simulink model "Final_IHA_2706_2015a"  (R2016b)
settings: Solver=ode5  StartTime=0.0  StopTime=20  FixedStep=SampleTime  RelTol=1e-3  EnableMultiTasking=on
values from neighbouring files (symbols this model uses):
  K = 2000    [code_final.m]
  PowerOn = 0    [code_final.m]
  q = 41.3    [code_final.m]
  Q_AT_break = [-1 -0.7 -0.5 -0.3 -0.2 -0.1 0 0.2 0.8 1]    [code_final.m]
  Q_AT_look = [1 0.1991 0.1227 0.07575 0.04002 0.01761 0.00075 5.86e-8 5.86e-8 5.86e-8]    [code_final.m]
  Q_BT_break = [-1 -0.6 -0.2 0 0.1 0.2 0.3 0.4 0.5 1]    [code_final.m]
  Q_BT_look = [5.86e-8 5.86e-8 5.86e-8 0.000913 0.02175 0.040 0.081 0.10 0.20 1]    [code_final.m]
  Q_PA_break = [-1 -0.6 -0.2 0 0.1 0.2 0.3 0.4 0.5 1]    [code_final.m]
  Q_PA_look = [5.86e-8 5.86e-8 5.86e-8 0.000876 0.0214 0.044 0.071 0.1 0.15 1]    [code_final.m]
  Q_PB_break = [-1 -0.7 -0.5 -0.3 -0.2 -0.1 0 0.2 0.8 1]    [code_final.m]
  Q_PB_look = [1 0.1498 0.1 0.077 0.03591 0.021 0.00082 5.86e-8 5.86e-8 5.86e-8]    [code_final.m]
  SampleTime = .001    (= 0.001)    [code_final.m]
undefined symbols (not defined in the file or in its folder): b, Cylinder, Cylinder1, Cylinder2, Cylinder3, Cylinder4, DiscIntNeverNeededParam, FC, FL1, FL2, FS, Lift, Pillar, Pinion, Piston, Rack, tilt, Valve, VS, X, X1, X2, Y, Z
undefined symbols (not defined in the file): Cyl, HoseA, HoseB, Valve2, Valve3, Valve4
libraries: sm_lib x67, simulink x32, nesl_utility x20, simulink_extras x3, xpcrtudplib x2, xpcobsoletelib x2
(part 3 of 4)

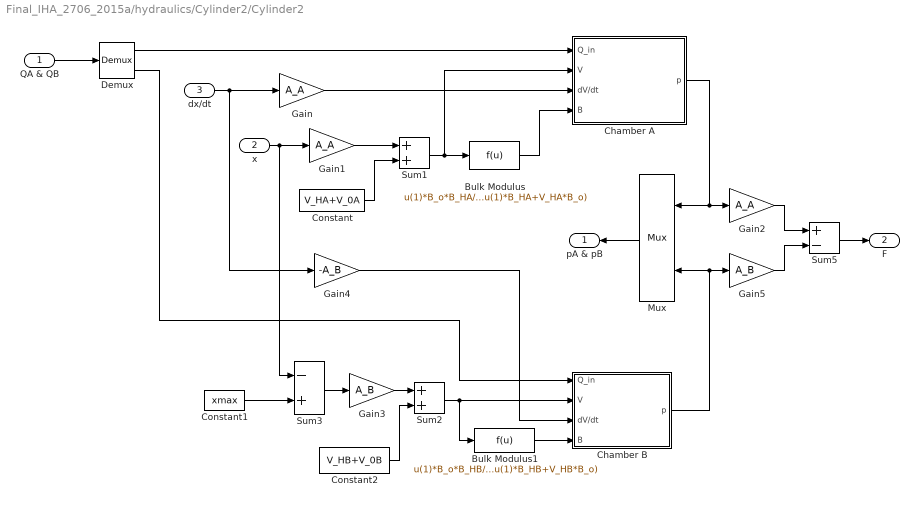
== system Final_IHA_2706_2015a/hydraulics/Cylinder2/Cylinder2 ==
  QA & QB : Inport
  x : Inport  Port=2
  dx/dt : Inport  Port=3
  Bulk Modulus : Fcn  Expr=u(1)*B_o*B_HA/(u(1)*B_HA+V_HA*B_o)
  Bulk Modulus1 : Fcn  Expr=u(1)*B_o*B_HB/(u(1)*B_HB+V_HB*B_o)
  Chamber A : Subsystem  mask(Hydraulic){pinitial=p_0A}
      mask prompts: pinitial "Initial pressure [Pa] :"
      mask help: Lumped fluid volume. Pressure is limited greater or equal to zero by saturation block corresponding to a rough model of cavitation.
      mask Help: eval('hydlibdoc(''vol_cav_doc'')')
  Chamber B : Subsystem  mask(Hydraulic){pinitial=p_0B}
      mask prompts: pinitial "Initial pressure [Pa] :"
      mask help: Lumped fluid volume. Pressure is limited greater or equal to zero by saturation block corresponding to a rough model of cavitation.
      mask Help: eval('hydlibdoc(''vol_cav_doc'')')
  Constant : Constant  Value=V_HA+V_0A
  Constant1 : Constant  Value=xmax
  Constant2 : Constant  Value=V_HB+V_0B
  Demux : Demux  Outputs=2
  Gain : Gain  Gain=A_A  SaturateOnIntegerOverflow=on  OutDataTypeStr=Inherit: Same as input  ParamDataTypeStr=Inherit: Same as input
  Gain1 : Gain  Gain=A_A  SaturateOnIntegerOverflow=on  OutDataTypeStr=Inherit: Same as input  ParamDataTypeStr=Inherit: Same as input
  Gain2 : Gain  Gain=A_A  SaturateOnIntegerOverflow=on  OutDataTypeStr=Inherit: Same as input  ParamDataTypeStr=Inherit: Same as input
  Gain3 : Gain  Gain=A_B  SaturateOnIntegerOverflow=on  OutDataTypeStr=Inherit: Same as input  ParamDataTypeStr=Inherit: Same as input
  Gain4 : Gain  Gain=-A_B  SaturateOnIntegerOverflow=on  OutDataTypeStr=Inherit: Same as input  ParamDataTypeStr=Inherit: Same as input
  Gain5 : Gain  Gain=A_B  SaturateOnIntegerOverflow=on  OutDataTypeStr=Inherit: Same as input  ParamDataTypeStr=Inherit: Same as input
  Mux : Mux  Inputs=2
  Sum1 : Sum  SaturateOnIntegerOverflow=on  InputSameDT=on  OutDataTypeStr=Inherit: Same as first input
  Sum2 : Sum  SaturateOnIntegerOverflow=on  InputSameDT=on  OutDataTypeStr=Inherit: Same as first input
  Sum3 : Sum  Inputs=-+  SaturateOnIntegerOverflow=on  InputSameDT=on  OutDataTypeStr=Inherit: Same as first input
  Sum5 : Sum  Inputs=+-  SaturateOnIntegerOverflow=on  InputSameDT=on  OutDataTypeStr=Inherit: Same as first input
  pA & pB : Outport  InitialOutput=0
  F : Outport  Port=2  InitialOutput=0
  wires:
  Constant/1 -> Sum1/2
  Sum1/1 -> Chamber A/2(" V"), Bulk Modulus/1
  Gain1/1 -> Sum1/1
  x/1 -> Gain1/1, Sum3/1
  QA & QB/1 -> Demux/1
  Chamber B/1(p) -> Gain5/1, Mux/2
  Sum5/1 -> F/1
  Gain5/1 -> Sum5/2
  Gain2/1 -> Sum5/1
  Chamber A/1(p) -> Gain2/1, Mux/1
  Mux/1 -> pA & pB/1
  Bulk Modulus/1 -> Chamber A/4(" B")
  Demux/1 -> Chamber A/1(Q_in)
  Bulk Modulus1/1 -> Chamber B/4(" B")
  Gain4/1 -> Chamber B/3(" dV/dt")
  Sum2/1 -> Chamber B/2(" V"), Bulk Modulus1/1
  Demux/2 -> Chamber B/1(Q_in)
  Constant1/1 -> Sum3/2
  Sum3/1 -> Gain3/1
  Gain3/1 -> Sum2/1
  Constant2/1 -> Sum2/2
  Gain/1 -> Chamber A/3(" dV/dt")
  dx/dt/1 -> Gain/1, Gain4/1

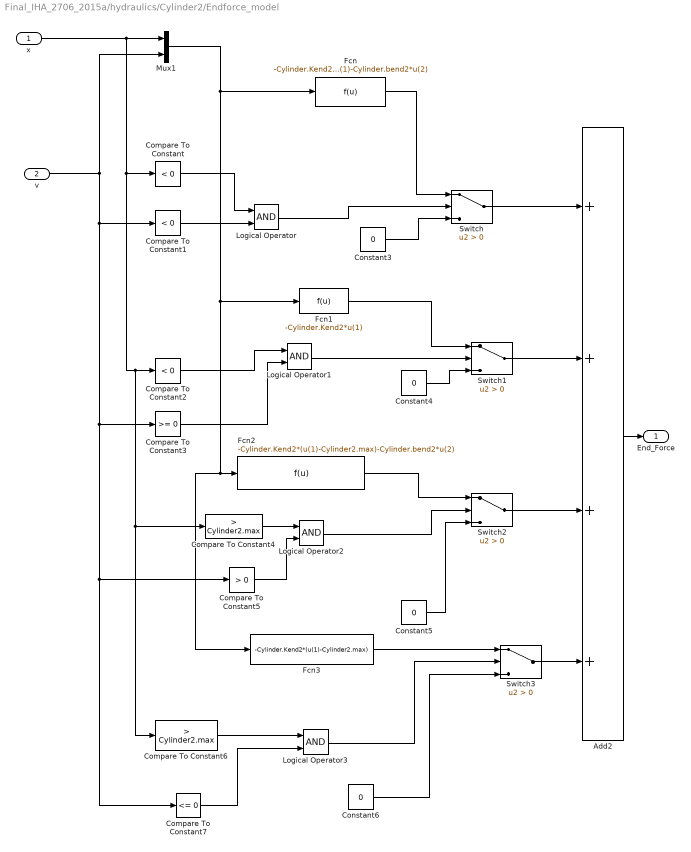
== system Final_IHA_2706_2015a/hydraulics/Cylinder2/Endforce_model ==
  x : Inport
  v : Inport  Port=2
  Add2 : Sum  Inputs=++++
  Compare To Constant : simulink/Logic and Bit Operations/Compare To Constant  relop=<  const=0  OutDataTypeStr=boolean
  Compare To Constant1 : simulink/Logic and Bit Operations/Compare To Constant  relop=<  const=0  OutDataTypeStr=boolean
  Compare To Constant2 : simulink/Logic and Bit Operations/Compare To Constant  relop=<  const=0  OutDataTypeStr=boolean
  Compare To Constant3 : simulink/Logic and Bit Operations/Compare To Constant  relop=>=  const=0  OutDataTypeStr=boolean
  Compare To Constant4 : simulink/Logic and Bit Operations/Compare To Constant  relop=>  const=Cylinder2.max  OutDataTypeStr=boolean
  Compare To Constant5 : simulink/Logic and Bit Operations/Compare To Constant  relop=>  const=0  OutDataTypeStr=boolean
  Compare To Constant6 : simulink/Logic and Bit Operations/Compare To Constant  relop=>  const=Cylinder2.max  OutDataTypeStr=boolean
  Compare To Constant7 : simulink/Logic and Bit Operations/Compare To Constant  relop=<=  const=0  OutDataTypeStr=boolean
  Constant{3..6} (4 alike) : Constant  Value=0
  Fcn : Fcn  Expr=-Cylinder.Kend2*u(1)-Cylinder.bend2*u(2)
  Fcn1 : Fcn  Expr=-Cylinder.Kend2*u(1)
  Fcn2 : Fcn  Expr=-Cylinder.Kend2*(u(1)-Cylinder2.max)-Cylinder.bend2*u(2)
  Fcn3 : Fcn  Expr=-Cylinder.Kend2*(u(1)-Cylinder2.max)
  Logical Operator{,1..3} (4 alike) : Logic  AllPortsSameDT=off  OutDataTypeStr=boolean
  Mux1 : Mux  Inputs=2
  Switch{,1..3} (4 alike) : Switch  Criteria=u2 > Threshold
  End_Force : Outport
  wires:
  x/1 -> Compare To Constant/1, Compare To Constant2/1, Compare To Constant4/1, Compare To Constant6/1, Mux1/1
  v/1 -> Compare To Constant1/1, Compare To Constant3/1, Compare To Constant5/1, Compare To Constant7/1, Mux1/2
  Fcn2/1 -> Switch2/1
  Logical Operator3/1 -> Switch3/2
  Fcn3/1 -> Switch3/1
  Compare To Constant5/1 -> Logical Operator2/2
  Switch2/1 -> Add2/3
  Constant6/1 -> Switch3/3
  Compare To Constant6/1 -> Logical Operator3/1
  Switch/1 -> Add2/1
  Constant5/1 -> Switch2/3
  Logical Operator2/1 -> Switch2/2
  Compare To Constant7/1 -> Logical Operator3/2
  Switch1/1 -> Add2/2
  Add2/1 -> End_Force/1
  Mux1/1 -> Fcn/1, Fcn3/1, Fcn2/1, Fcn1/1
  Switch3/1 -> Add2/4
  Compare To Constant2/1 -> Logical Operator1/1
  Compare To Constant1/1 -> Logical Operator/2
  Constant4/1 -> Switch1/3
  Logical Operator1/1 -> Switch1/2
  Fcn/1 -> Switch/1
  Logical Operator/1 -> Switch/2
  Constant3/1 -> Switch/3
  Compare To Constant/1 -> Logical Operator/1
  Compare To Constant4/1 -> Logical Operator2/1
  Fcn1/1 -> Switch1/1
  Compare To Constant3/1 -> Logical Operator1/2

== system Final_IHA_2706_2015a/hydraulics/Cylinder2/Friction_model ==
  v : Inport
  Add : Sum
  Fcn : Fcn  Expr=tanh(K*u)
  Fcn1 : Fcn  Expr=FC.c2+(FS.c2-FC.c2)*exp(-(u/VS.c2)^2)
  Fcn2 : Fcn  Expr=b.c2*u
  Product : Product
  Friction_Force : Outport
  wires:
  Fcn/1 -> Product/1
  Fcn1/1 -> Product/2
  Fcn2/1 -> Add/2
  Product/1 -> Add/1
  v/1 -> Fcn/1, Fcn2/1, Fcn1/1
  Add/1 -> Friction_Force/1

== system Final_IHA_2706_2015a/hydraulics/Cylinder2/Valve System2 ==
  p_A : Inport
  Uvalve : Inport  Port=2
  p_B : Inport  Port=3
  p_S : Inport  Port=4
  p_T : Inport  Port=5
  Flow paths : Subsystem
  Relative openings : Subsystem
  Scope : Scope
  Terminator1 : Terminator
  Terminator2 : Terminator
  Valve Dynamics : Subsystem
  Q_A : Outport
  Q_B : Outport  Port=2
  wires:
  p_A/1 -> Flow paths/5(p_A)
  p_T/1 -> Flow paths/8("p_T ")
  p_S/1 -> Flow paths/7(p_S)
  Flow paths/1(Q_A) -> Q_A/1, Scope/1
  p_B/1 -> Flow paths/6(p_B)
  Relative openings/1(av_PA) -> Flow paths/1(av_PA)
  Relative openings/3(av_BT) -> Flow paths/2(av_BT)
  Relative openings/4(av_AT) -> Flow paths/4(av_AT)
  Relative openings/2(av_PB) -> Flow paths/3(av_PB)
  Valve Dynamics/1(Spool Position [-1....1]) -> Relative openings/1(Spool_position)
  Flow paths/4(Q_T) -> Terminator2/1
  Flow paths/3(Q_P) -> Terminator1/1
  Flow paths/2(Q_B) -> Q_B/1
  Uvalve/1 -> Valve Dynamics/1(Control [-1....1])

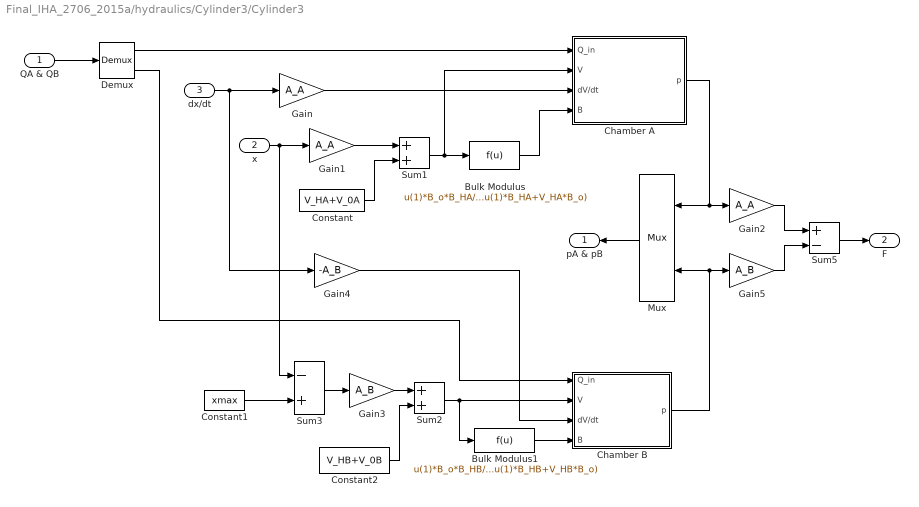
== system Final_IHA_2706_2015a/hydraulics/Cylinder3/Cylinder3 ==
  QA & QB : Inport
  x : Inport  Port=2
  dx/dt : Inport  Port=3
  Bulk Modulus : Fcn  Expr=u(1)*B_o*B_HA/(u(1)*B_HA+V_HA*B_o)
  Bulk Modulus1 : Fcn  Expr=u(1)*B_o*B_HB/(u(1)*B_HB+V_HB*B_o)
  Chamber A : Subsystem  mask(Hydraulic){pinitial=p_0A}
      mask prompts: pinitial "Initial pressure [Pa] :"
      mask help: Lumped fluid volume. Pressure is limited greater or equal to zero by saturation block corresponding to a rough model of cavitation.
      mask Help: eval('hydlibdoc(''vol_cav_doc'')')
  Chamber B : Subsystem  mask(Hydraulic){pinitial=p_0B}
      mask prompts: pinitial "Initial pressure [Pa] :"
      mask help: Lumped fluid volume. Pressure is limited greater or equal to zero by saturation block corresponding to a rough model of cavitation.
      mask Help: eval('hydlibdoc(''vol_cav_doc'')')
  Constant : Constant  Value=V_HA+V_0A
  Constant1 : Constant  Value=xmax
  Constant2 : Constant  Value=V_HB+V_0B
  Demux : Demux  Outputs=2
  Gain : Gain  Gain=A_A  SaturateOnIntegerOverflow=on  OutDataTypeStr=Inherit: Same as input  ParamDataTypeStr=Inherit: Same as input
  Gain1 : Gain  Gain=A_A  SaturateOnIntegerOverflow=on  OutDataTypeStr=Inherit: Same as input  ParamDataTypeStr=Inherit: Same as input
  Gain2 : Gain  Gain=A_A  SaturateOnIntegerOverflow=on  OutDataTypeStr=Inherit: Same as input  ParamDataTypeStr=Inherit: Same as input
  Gain3 : Gain  Gain=A_B  SaturateOnIntegerOverflow=on  OutDataTypeStr=Inherit: Same as input  ParamDataTypeStr=Inherit: Same as input
  Gain4 : Gain  Gain=-A_B  SaturateOnIntegerOverflow=on  OutDataTypeStr=Inherit: Same as input  ParamDataTypeStr=Inherit: Same as input
  Gain5 : Gain  Gain=A_B  SaturateOnIntegerOverflow=on  OutDataTypeStr=Inherit: Same as input  ParamDataTypeStr=Inherit: Same as input
  Mux : Mux  Inputs=2
  Sum1 : Sum  SaturateOnIntegerOverflow=on  InputSameDT=on  OutDataTypeStr=Inherit: Same as first input
  Sum2 : Sum  SaturateOnIntegerOverflow=on  InputSameDT=on  OutDataTypeStr=Inherit: Same as first input
  Sum3 : Sum  Inputs=-+  SaturateOnIntegerOverflow=on  InputSameDT=on  OutDataTypeStr=Inherit: Same as first input
  Sum5 : Sum  Inputs=+-  SaturateOnIntegerOverflow=on  InputSameDT=on  OutDataTypeStr=Inherit: Same as first input
  pA & pB : Outport  InitialOutput=0
  F : Outport  Port=2  InitialOutput=0
  wires:
  dx/dt/1 -> Gain4/1, Gain/1
  Gain/1 -> Chamber A/3(" dV/dt")
  Constant2/1 -> Sum2/2
  Gain3/1 -> Sum2/1
  Sum3/1 -> Gain3/1
  Constant1/1 -> Sum3/2
  Demux/2 -> Chamber B/1(Q_in)
  Sum2/1 -> Bulk Modulus1/1, Chamber B/2(" V")
  Gain4/1 -> Chamber B/3(" dV/dt")
  Bulk Modulus1/1 -> Chamber B/4(" B")
  Demux/1 -> Chamber A/1(Q_in)
  Bulk Modulus/1 -> Chamber A/4(" B")
  Mux/1 -> pA & pB/1
  Chamber A/1(p) -> Mux/1, Gain2/1
  Gain2/1 -> Sum5/1
  Gain5/1 -> Sum5/2
  Sum5/1 -> F/1
  Chamber B/1(p) -> Mux/2, Gain5/1
  QA & QB/1 -> Demux/1
  x/1 -> Sum3/1, Gain1/1
  Gain1/1 -> Sum1/1
  Sum1/1 -> Bulk Modulus/1, Chamber A/2(" V")
  Constant/1 -> Sum1/2

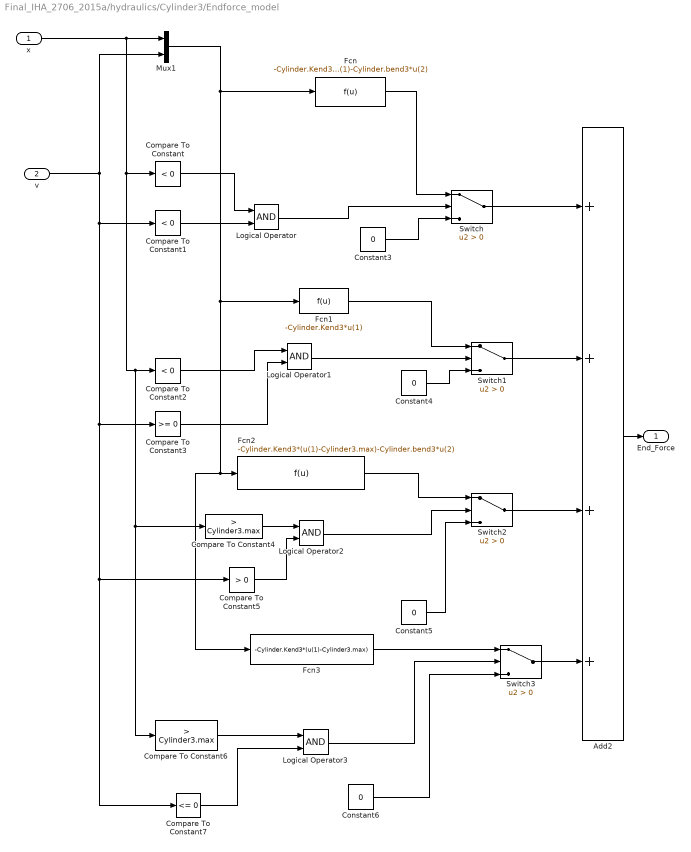
== system Final_IHA_2706_2015a/hydraulics/Cylinder3/Endforce_model ==
  x : Inport
  v : Inport  Port=2
  Add2 : Sum  Inputs=++++
  Compare To Constant : simulink/Logic and Bit Operations/Compare To Constant  relop=<  const=0  OutDataTypeStr=boolean
  Compare To Constant1 : simulink/Logic and Bit Operations/Compare To Constant  relop=<  const=0  OutDataTypeStr=boolean
  Compare To Constant2 : simulink/Logic and Bit Operations/Compare To Constant  relop=<  const=0  OutDataTypeStr=boolean
  Compare To Constant3 : simulink/Logic and Bit Operations/Compare To Constant  relop=>=  const=0  OutDataTypeStr=boolean
  Compare To Constant4 : simulink/Logic and Bit Operations/Compare To Constant  relop=>  const=Cylinder3.max  OutDataTypeStr=boolean
  Compare To Constant5 : simulink/Logic and Bit Operations/Compare To Constant  relop=>  const=0  OutDataTypeStr=boolean
  Compare To Constant6 : simulink/Logic and Bit Operations/Compare To Constant  relop=>  const=Cylinder3.max  OutDataTypeStr=boolean
  Compare To Constant7 : simulink/Logic and Bit Operations/Compare To Constant  relop=<=  const=0  OutDataTypeStr=boolean
  Constant{3..6} (4 alike) : Constant  Value=0
  Fcn : Fcn  Expr=-Cylinder.Kend3*u(1)-Cylinder.bend3*u(2)
  Fcn1 : Fcn  Expr=-Cylinder.Kend3*u(1)
  Fcn2 : Fcn  Expr=-Cylinder.Kend3*(u(1)-Cylinder3.max)-Cylinder.bend3*u(2)
  Fcn3 : Fcn  Expr=-Cylinder.Kend3*(u(1)-Cylinder3.max)
  Logical Operator{,1..3} (4 alike) : Logic  AllPortsSameDT=off  OutDataTypeStr=boolean
  Mux1 : Mux  Inputs=2
  Switch{,1..3} (4 alike) : Switch  Criteria=u2 > Threshold
  End_Force : Outport
  wires:
  Compare To Constant3/1 -> Logical Operator1/2
  Fcn1/1 -> Switch1/1
  Compare To Constant4/1 -> Logical Operator2/1
  Compare To Constant/1 -> Logical Operator/1
  Constant3/1 -> Switch/3
  Logical Operator/1 -> Switch/2
  Fcn/1 -> Switch/1
  Logical Operator1/1 -> Switch1/2
  Constant4/1 -> Switch1/3
  Compare To Constant1/1 -> Logical Operator/2
  Compare To Constant2/1 -> Logical Operator1/1
  Switch3/1 -> Add2/4
  Mux1/1 -> Fcn1/1, Fcn2/1, Fcn3/1, Fcn/1
  Add2/1 -> End_Force/1
  Switch1/1 -> Add2/2
  Compare To Constant7/1 -> Logical Operator3/2
  Logical Operator2/1 -> Switch2/2
  Constant5/1 -> Switch2/3
  Switch/1 -> Add2/1
  Compare To Constant6/1 -> Logical Operator3/1
  Constant6/1 -> Switch3/3
  Switch2/1 -> Add2/3
  Compare To Constant5/1 -> Logical Operator2/2
  Fcn3/1 -> Switch3/1
  Logical Operator3/1 -> Switch3/2
  Fcn2/1 -> Switch2/1
  v/1 -> Mux1/2, Compare To Constant7/1, Compare To Constant5/1, Compare To Constant3/1, Compare To Constant1/1
  x/1 -> Mux1/1, Compare To Constant6/1, Compare To Constant4/1, Compare To Constant2/1, Compare To Constant/1

== system Final_IHA_2706_2015a/hydraulics/Cylinder3/Friction_model ==
  v : Inport
  Add : Sum
  Fcn : Fcn  Expr=tanh(K*u)
  Fcn1 : Fcn  Expr=FC.c3+(FS.c3-FC.c3)*exp(-(u/VS.c3)^2)
  Fcn2 : Fcn  Expr=b.c3*u
  Product : Product
  Friction_Force : Outport
  wires:
  Add/1 -> Friction_Force/1
  v/1 -> Fcn1/1, Fcn2/1, Fcn/1
  Product/1 -> Add/1
  Fcn2/1 -> Add/2
  Fcn1/1 -> Product/2
  Fcn/1 -> Product/1

== system Final_IHA_2706_2015a/hydraulics/Cylinder3/Valve System3 ==
  p_A : Inport
  Uvalve : Inport  Port=2
  p_B : Inport  Port=3
  p_S : Inport  Port=4
  p_T : Inport  Port=5
  Flow paths : Subsystem
  Relative openings : Subsystem
  Scope : Scope
  Terminator1 : Terminator
  Terminator2 : Terminator
  Valve Dynamics : Subsystem
  Q_A : Outport
  Q_B : Outport  Port=2
  wires:
  Uvalve/1 -> Valve Dynamics/1(Control [-1....1])
  Flow paths/2(Q_B) -> Q_B/1
  Flow paths/3(Q_P) -> Terminator1/1
  Flow paths/4(Q_T) -> Terminator2/1
  Valve Dynamics/1(Spool Position [-1....1]) -> Relative openings/1(Spool_position)
  Relative openings/2(av_PB) -> Flow paths/3(av_PB)
  Relative openings/4(av_AT) -> Flow paths/4(av_AT)
  Relative openings/3(av_BT) -> Flow paths/2(av_BT)
  Relative openings/1(av_PA) -> Flow paths/1(av_PA)
  p_B/1 -> Flow paths/6(p_B)
  Flow paths/1(Q_A) -> Scope/1, Q_A/1
  p_S/1 -> Flow paths/7(p_S)
  p_T/1 -> Flow paths/8("p_T ")
  p_A/1 -> Flow paths/5(p_A)

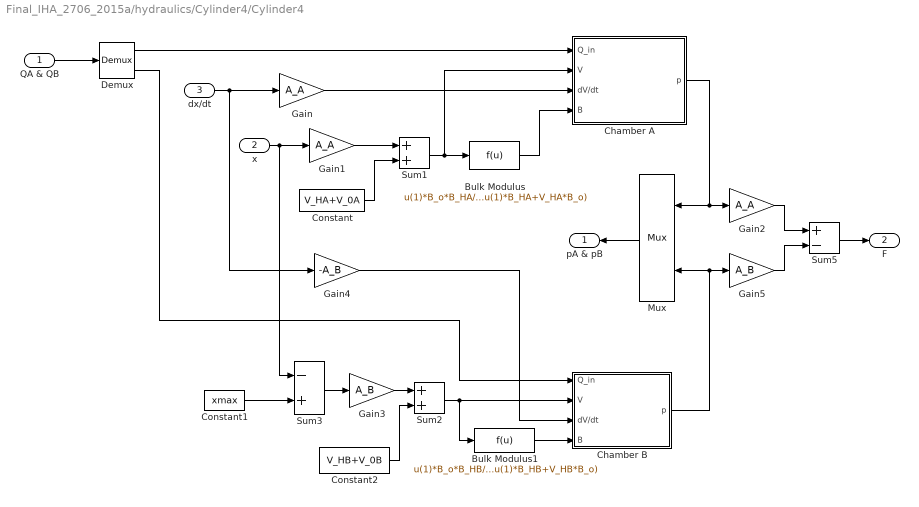
== system Final_IHA_2706_2015a/hydraulics/Cylinder4/Cylinder4 ==
  QA & QB : Inport
  x : Inport  Port=2
  dx/dt : Inport  Port=3
  Bulk Modulus : Fcn  Expr=u(1)*B_o*B_HA/(u(1)*B_HA+V_HA*B_o)
  Bulk Modulus1 : Fcn  Expr=u(1)*B_o*B_HB/(u(1)*B_HB+V_HB*B_o)
  Chamber A : Subsystem  mask(Hydraulic){pinitial=p_0A}
      mask prompts: pinitial "Initial pressure [Pa] :"
      mask help: Lumped fluid volume. Pressure is limited greater or equal to zero by saturation block corresponding to a rough model of cavitation.
      mask Help: eval('hydlibdoc(''vol_cav_doc'')')
  Chamber B : Subsystem  mask(Hydraulic){pinitial=p_0B}
      mask prompts: pinitial "Initial pressure [Pa] :"
      mask help: Lumped fluid volume. Pressure is limited greater or equal to zero by saturation block corresponding to a rough model of cavitation.
      mask Help: eval('hydlibdoc(''vol_cav_doc'')')
  Constant : Constant  Value=V_HA+V_0A
  Constant1 : Constant  Value=xmax
  Constant2 : Constant  Value=V_HB+V_0B
  Demux : Demux  Outputs=2
  Gain : Gain  Gain=A_A  SaturateOnIntegerOverflow=on  OutDataTypeStr=Inherit: Same as input  ParamDataTypeStr=Inherit: Same as input
  Gain1 : Gain  Gain=A_A  SaturateOnIntegerOverflow=on  OutDataTypeStr=Inherit: Same as input  ParamDataTypeStr=Inherit: Same as input
  Gain2 : Gain  Gain=A_A  SaturateOnIntegerOverflow=on  OutDataTypeStr=Inherit: Same as input  ParamDataTypeStr=Inherit: Same as input
  Gain3 : Gain  Gain=A_B  SaturateOnIntegerOverflow=on  OutDataTypeStr=Inherit: Same as input  ParamDataTypeStr=Inherit: Same as input
  Gain4 : Gain  Gain=-A_B  SaturateOnIntegerOverflow=on  OutDataTypeStr=Inherit: Same as input  ParamDataTypeStr=Inherit: Same as input
  Gain5 : Gain  Gain=A_B  SaturateOnIntegerOverflow=on  OutDataTypeStr=Inherit: Same as input  ParamDataTypeStr=Inherit: Same as input
  Mux : Mux  Inputs=2
  Sum1 : Sum  SaturateOnIntegerOverflow=on  InputSameDT=on  OutDataTypeStr=Inherit: Same as first input
  Sum2 : Sum  SaturateOnIntegerOverflow=on  InputSameDT=on  OutDataTypeStr=Inherit: Same as first input
  Sum3 : Sum  Inputs=-+  SaturateOnIntegerOverflow=on  InputSameDT=on  OutDataTypeStr=Inherit: Same as first input
  Sum5 : Sum  Inputs=+-  SaturateOnIntegerOverflow=on  InputSameDT=on  OutDataTypeStr=Inherit: Same as first input
  pA & pB : Outport  InitialOutput=0
  F : Outport  Port=2  InitialOutput=0
  wires:
  Constant/1 -> Sum1/2
  Sum1/1 -> Chamber A/2(" V"), Bulk Modulus/1
  Gain1/1 -> Sum1/1
  x/1 -> Gain1/1, Sum3/1
  QA & QB/1 -> Demux/1
  Chamber B/1(p) -> Gain5/1, Mux/2
  Sum5/1 -> F/1
  Gain5/1 -> Sum5/2
  Gain2/1 -> Sum5/1
  Chamber A/1(p) -> Gain2/1, Mux/1
  Mux/1 -> pA & pB/1
  Bulk Modulus/1 -> Chamber A/4(" B")
  Demux/1 -> Chamber A/1(Q_in)
  Bulk Modulus1/1 -> Chamber B/4(" B")
  Gain4/1 -> Chamber B/3(" dV/dt")
  Sum2/1 -> Chamber B/2(" V"), Bulk Modulus1/1
  Demux/2 -> Chamber B/1(Q_in)
  Constant1/1 -> Sum3/2
  Sum3/1 -> Gain3/1
  Gain3/1 -> Sum2/1
  Constant2/1 -> Sum2/2
  Gain/1 -> Chamber A/3(" dV/dt")
  dx/dt/1 -> Gain/1, Gain4/1

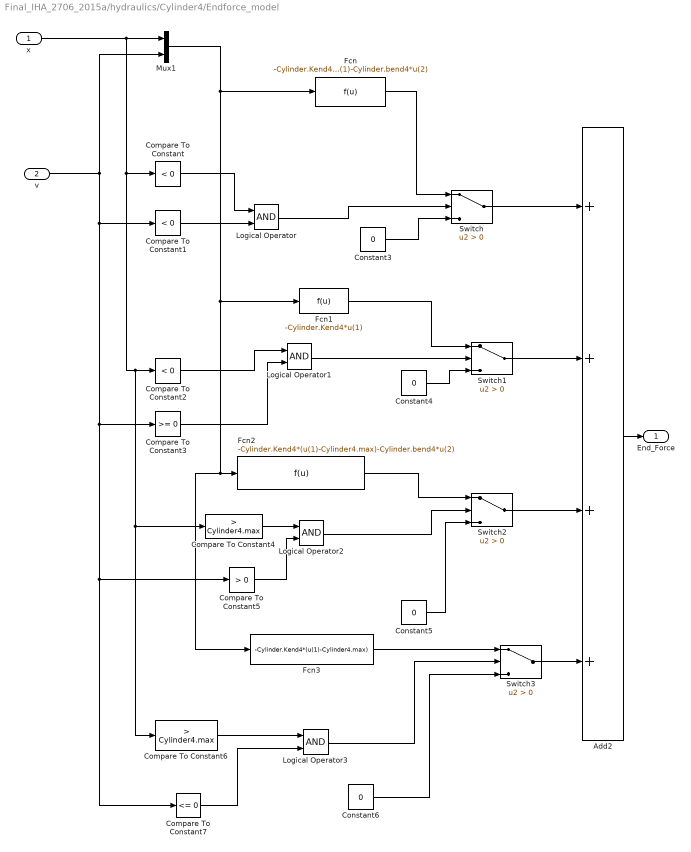
== system Final_IHA_2706_2015a/hydraulics/Cylinder4/Endforce_model ==
  x : Inport
  v : Inport  Port=2
  Add2 : Sum  Inputs=++++
  Compare To Constant : simulink/Logic and Bit Operations/Compare To Constant  relop=<  const=0  OutDataTypeStr=boolean
  Compare To Constant1 : simulink/Logic and Bit Operations/Compare To Constant  relop=<  const=0  OutDataTypeStr=boolean
  Compare To Constant2 : simulink/Logic and Bit Operations/Compare To Constant  relop=<  const=0  OutDataTypeStr=boolean
  Compare To Constant3 : simulink/Logic and Bit Operations/Compare To Constant  relop=>=  const=0  OutDataTypeStr=boolean
  Compare To Constant4 : simulink/Logic and Bit Operations/Compare To Constant  relop=>  const=Cylinder4.max  OutDataTypeStr=boolean
  Compare To Constant5 : simulink/Logic and Bit Operations/Compare To Constant  relop=>  const=0  OutDataTypeStr=boolean
  Compare To Constant6 : simulink/Logic and Bit Operations/Compare To Constant  relop=>  const=Cylinder4.max  OutDataTypeStr=boolean
  Compare To Constant7 : simulink/Logic and Bit Operations/Compare To Constant  relop=<=  const=0  OutDataTypeStr=boolean
  Constant{3..6} (4 alike) : Constant  Value=0
  Fcn : Fcn  Expr=-Cylinder.Kend4*u(1)-Cylinder.bend4*u(2)
  Fcn1 : Fcn  Expr=-Cylinder.Kend4*u(1)
  Fcn2 : Fcn  Expr=-Cylinder.Kend4*(u(1)-Cylinder4.max)-Cylinder.bend4*u(2)
  Fcn3 : Fcn  Expr=-Cylinder.Kend4*(u(1)-Cylinder4.max)
  Logical Operator{,1..3} (4 alike) : Logic  AllPortsSameDT=off  OutDataTypeStr=boolean
  Mux1 : Mux  Inputs=2
  Switch{,1..3} (4 alike) : Switch  Criteria=u2 > Threshold
  End_Force : Outport
  wires:
  x/1 -> Compare To Constant/1, Compare To Constant2/1, Compare To Constant4/1, Compare To Constant6/1, Mux1/1
  v/1 -> Compare To Constant1/1, Compare To Constant3/1, Compare To Constant5/1, Compare To Constant7/1, Mux1/2
  Fcn2/1 -> Switch2/1
  Logical Operator3/1 -> Switch3/2
  Fcn3/1 -> Switch3/1
  Compare To Constant5/1 -> Logical Operator2/2
  Switch2/1 -> Add2/3
  Constant6/1 -> Switch3/3
  Compare To Constant6/1 -> Logical Operator3/1
  Switch/1 -> Add2/1
  Constant5/1 -> Switch2/3
  Logical Operator2/1 -> Switch2/2
  Compare To Constant7/1 -> Logical Operator3/2
  Switch1/1 -> Add2/2
  Add2/1 -> End_Force/1
  Mux1/1 -> Fcn/1, Fcn3/1, Fcn2/1, Fcn1/1
  Switch3/1 -> Add2/4
  Compare To Constant2/1 -> Logical Operator1/1
  Compare To Constant1/1 -> Logical Operator/2
  Constant4/1 -> Switch1/3
  Logical Operator1/1 -> Switch1/2
  Fcn/1 -> Switch/1
  Logical Operator/1 -> Switch/2
  Constant3/1 -> Switch/3
  Compare To Constant/1 -> Logical Operator/1
  Compare To Constant4/1 -> Logical Operator2/1
  Fcn1/1 -> Switch1/1
  Compare To Constant3/1 -> Logical Operator1/2

== system Final_IHA_2706_2015a/hydraulics/Cylinder4/Friction_model ==
  v : Inport
  Add : Sum
  Fcn : Fcn  Expr=tanh(K*u)
  Fcn1 : Fcn  Expr=FC.c3+(FS.c3-FC.c3)*exp(-(u/VS.c3)^2)
  Fcn2 : Fcn  Expr=b.c3*u
  Product : Product
  Friction_Force : Outport
  wires:
  Fcn/1 -> Product/1
  Fcn1/1 -> Product/2
  Fcn2/1 -> Add/2
  Product/1 -> Add/1
  v/1 -> Fcn/1, Fcn2/1, Fcn1/1
  Add/1 -> Friction_Force/1

== system Final_IHA_2706_2015a/hydraulics/Cylinder4/Valve System4 ==
  p_A : Inport
  Uvalve : Inport  Port=2
  p_B : Inport  Port=3
  p_S : Inport  Port=4
  p_T : Inport  Port=5
  Flow paths : Subsystem
  Relative openings : Subsystem
  Scope : Scope
  Terminator1 : Terminator
  Terminator2 : Terminator
  Valve Dynamics : Subsystem
  Q_A : Outport
  Q_B : Outport  Port=2
  wires:
  p_A/1 -> Flow paths/5(p_A)
  p_T/1 -> Flow paths/8("p_T ")
  p_S/1 -> Flow paths/7(p_S)
  Flow paths/1(Q_A) -> Q_A/1, Scope/1
  p_B/1 -> Flow paths/6(p_B)
  Relative openings/1(av_PA) -> Flow paths/1(av_PA)
  Relative openings/3(av_BT) -> Flow paths/2(av_BT)
  Relative openings/4(av_AT) -> Flow paths/4(av_AT)
  Relative openings/2(av_PB) -> Flow paths/3(av_PB)
  Valve Dynamics/1(Spool Position [-1....1]) -> Relative openings/1(Spool_position)
  Flow paths/4(Q_T) -> Terminator2/1
  Flow paths/3(Q_P) -> Terminator1/1
  Flow paths/2(Q_B) -> Q_B/1
  Uvalve/1 -> Valve Dynamics/1(Control [-1....1])

== system Final_IHA_2706_2015a/manipulator/Extrusion 1 and 2/X1 ==
  Discrete-Time Integrator : DiscreteIntegrator  InitialConditionSetting=State (most efficient)  SampleTime=SampleTime  ICPrevOutput=DiscIntNeverNeededParam  ICPrevScaledInput=DiscIntNeverNeededParam
  PS-Simulink Converter2 : nesl_utility/PS-Simulink Converter  PhysicalDomain=network_engine_domain  SubClassName=ps_output  LeftPortType=input  RightPortType=output  PseudoPeriodic=off  Frequencies=[]  Unit=1  AffineConversion=off
  Prismatic Joint : sm_lib/Joints/Prismatic Joint  SenseConstraintForce=off  SenseConstraintForceX=off  SenseConstraintForceY=off  SenseConstraintForceZ=off  SenseConstraintTorque=off  SenseConstraintTorqueX=off  SenseConstraintTorqueY=off  SenseConstraintTorqueZ=off  SenseTotalForce=off  SenseTotalForceX=off  SenseTotalForceY=off  SenseTotalForceZ=off  SenseTotalTorque=off  SenseTotalTorqueX=off  SenseTotalTorqueY=off  SenseTotalTorqueZ=off  CompositeWrenchDir=FollowerOnBase  CompositeWrenchFrame=BaseFrame  EquilibriumPosition=0  EquilibriumPositionUnits=m  SpringStiffness=0  SpringStiffnessUnits=N/m  DampingCoefficient=0  DampingCoefficientUnits=N/(m/s)  TorqueActuationMode=NoTorque  MotionActuationMode=ComputedMotion  SensePosition=off  SenseVelocity=on  SenseAcceleration=off  SenseTorqueForce=off  PositionTargetSpecify=off  PositionTargetPriority=High  PositionTargetValue=0  PositionTargetValueUnits=m  VelocityTargetSpecify=off  VelocityTargetPriority=High  VelocityTargetValue=0  VelocityTargetValueUnits=m/s
  Rigid Transform : sm_lib/Frames and Transforms/Rigid Transform  TranslationMethod=None  TranslationStandardOffset=X1.pos  TranslationLengthUnit=m  TranslationStandardAxis=-X  TranslationCartesianOffset=[0 0 0]  TranslationROffset=0  TranslationROffsetUnits=m  TranslationZOffset=0  TranslationZOffsetUnits=m  TranslationThetaOffset=0  TranslationThetaOffsetUnits=deg  RotationMethod=StandardAxis  RotationAngleUnits=deg  RotationStandardAxis=+Y  RotationAngle=-90  RotationArbitraryAxis=[0 0 1]  FollAlignAxisA=+X  BaseAlignAxisA=+Y  FollAlignAxisB=+Y  BaseAlignAxisB=+Z  RotationSequenceAxes=FollowerAxes  RotationSequence=XYX  RotationSequenceAngles=[0 0 0]  RotationSequenceAnglesUnits=deg  RotationMatrix=[1 0 0; 0 1 0; 0 0 1]
  Signal Conversion1 : SignalConversion  OverrideOpt=off
  Simulink-PS Converter : nesl_utility/Simulink-PS Converter  PhysicalDomain=network_engine_domain  SubClassName=ps_input  LeftPortType=input  RightPortType=output  PseudoPeriodic=off  Frequencies=[]  NoiseDistribution=none  NoiseParameters=[]  Unit=1  AffineConversion=off  InputFiltering=off  SimscapeFilterOrder=1  InputFilterTimeConstant=0.001  UdotUserProvided=1
  Terminator1 : Terminator
  X1 : sm_lib/Body Elements/Solid  InertiaType=Custom  Mass=X1.m  MassUnits=kg  CenterOfMass=X1.cm  CenterOfMassUnits=m  MomentsOfInertia=[1 1 1]  MomentsOfInertiaUnits=kg*m^2  ProductsOfInertia=[0 0 0]  ProductsOfInertiaUnits=kg*m^2  DensityBased=on  Density=1000  DensityUnits=kg/(m^3)  DoExposeReferenceFrame=on  SerializedFrames=<Frames/>  GraphicType=FromGeometry  MarkerShape=Sphere  MarkerSize=10  MarkerSizeUnits=m  GraphicVisPropType=SimpleVisualProperties  GraphicDiffuseColor=X1.rgb  GraphicSpecularColor=[0.5 0.5 0.5 1.0]  GraphicAmbientColor=[0.15 0.15 0.15 1.0]  GraphicEmissiveColor=[0.0 0.0 0.0 1.0]  GraphicShininess=75  GraphicOpacity=1.0  GeometryShape=GeneralExtrusion  RectangleSize=[1 1]  RectangleSizeUnits=m  BrickDimensions=[1 1 1]  BrickDimensionUnits=m  CylinderRadius=1  CylinderRadiusUnits=m  CylinderLength=1  CylinderLengthUnits=m  SphereRadius=1  SphereRadiusUnits=m  EllipsoidRadii=[1 1 1]  EllipsoidRadiiUnits=m  ExtrusionCrossSection=X1.c  ExtrusionCrossSectionUnits=m  ExtrusionLength=X1.l  ExtrusionLengthUnits=m  PolygonNumSides=3  PolygonOuterRadius=1  PolygonOuterRadiusUnits=m  ExtGeomFileType=STEP  ExtGeomFileUnits=m  RevolutionCrossSection=[1 1; 1 -1; 2 -1; 2 1]  RevolutionCrossSectionUnits=m  RevolutionExtent=Full  RevolutionAngle=180  RevolutionAngleUnits=deg
  X_v1 : Scope
  to Piston4 : sm_lib/Frames and Transforms/Rigid Transform  TranslationMethod=Cartesian  TranslationStandardOffset=0  TranslationLengthUnit=m  TranslationStandardAxis=+Z  TranslationCartesianOffset=Piston.pos4  TranslationROffset=0  TranslationROffsetUnits=m  TranslationZOffset=0  TranslationZOffsetUnits=m  TranslationThetaOffset=0  TranslationThetaOffsetUnits=deg  RotationMethod=None  RotationAngleUnits=deg  RotationStandardAxis=+Z  RotationAngle=0.0  RotationArbitraryAxis=[0 0 1]  FollAlignAxisA=+X  BaseAlignAxisA=+Y  FollAlignAxisB=+Y  BaseAlignAxisB=+Z  RotationSequenceAxes=FollowerAxes  RotationSequence=XYX  RotationSequenceAngles=[0 0 0]  RotationSequenceAnglesUnits=deg  RotationMatrix=[1 0 0; 0 1 0; 0 0 1]
  To Piston 4 : PMIOPort  Port=1  Side=Left
  To X1 : PMIOPort  Port=2  Side=Left
  to X2v : PMIOPort  Port=3  Side=Left
  From X1 : PMIOPort  Port=4  Side=Right
  wires:
  PS-Simulink Converter2/1 -> Signal Conversion1/1, Discrete-Time Integrator/1
  Discrete-Time Integrator/1 -> Simulink-PS Converter/1
  Signal Conversion1/1 -> X_v1/1, Terminator1/1
  connections:
  to X2v/RConn1 -- Simulink-PS Converter/RConn1
  Rigid Transform/LConn1 -- Prismatic Joint/RConn1
  To X1/RConn1 -- Prismatic Joint/LConn1
  X1/RConn1 -- From X1/RConn1 -- to Piston4/LConn1 -- Rigid Transform/RConn1
  To Piston 4/RConn1 -- to Piston4/RConn1
  Prismatic Joint/RConn2 -- PS-Simulink Converter2/LConn1

== system Final_IHA_2706_2015a/manipulator/Extrusion 1 and 2/X2 ==
  Cylinder Joint2 : sm_lib/Joints/Prismatic Joint  SenseConstraintForce=off  SenseConstraintForceX=off  SenseConstraintForceY=off  SenseConstraintForceZ=off  SenseConstraintTorque=off  SenseConstraintTorqueX=off  SenseConstraintTorqueY=off  SenseConstraintTorqueZ=off  SenseTotalForce=off  SenseTotalForceX=off  SenseTotalForceY=off  SenseTotalForceZ=off  SenseTotalTorque=off  SenseTotalTorqueX=off  SenseTotalTorqueY=off  SenseTotalTorqueZ=off  CompositeWrenchDir=FollowerOnBase  CompositeWrenchFrame=BaseFrame  EquilibriumPosition=0  EquilibriumPositionUnits=m  SpringStiffness=0  SpringStiffnessUnits=N/m  DampingCoefficient=0  DampingCoefficientUnits=N/(m/s)  TorqueActuationMode=ComputedTorque  MotionActuationMode=InputMotion  SensePosition=off  SenseVelocity=on  SenseAcceleration=off  SenseTorqueForce=off  PositionTargetSpecify=off  PositionTargetPriority=High  PositionTargetValue=0  PositionTargetValueUnits=m  VelocityTargetSpecify=off  VelocityTargetPriority=High  VelocityTargetValue=0  VelocityTargetValueUnits=m/s
  PS-Simulink Converter1 : nesl_utility/PS-Simulink Converter  PhysicalDomain=network_engine_domain  SubClassName=ps_output  LeftPortType=input  RightPortType=output  PseudoPeriodic=off  Frequencies=[]  Unit=1  AffineConversion=off
  Rigid Transform1 : sm_lib/Frames and Transforms/Rigid Transform  TranslationMethod=None  TranslationStandardOffset=0  TranslationLengthUnit=m  TranslationStandardAxis=+Z  TranslationCartesianOffset=[0 0 0]  TranslationROffset=0  TranslationROffsetUnits=m  TranslationZOffset=0  TranslationZOffsetUnits=m  TranslationThetaOffset=0  TranslationThetaOffsetUnits=deg  RotationMethod=StandardAxis  RotationAngleUnits=deg  RotationStandardAxis=+Y  RotationAngle=-90  RotationArbitraryAxis=[0 0 1]  FollAlignAxisA=+X  BaseAlignAxisA=+Y  FollAlignAxisB=+Y  BaseAlignAxisB=+Z  RotationSequenceAxes=FollowerAxes  RotationSequence=XYX  RotationSequenceAngles=[0 0 0]  RotationSequenceAnglesUnits=deg  RotationMatrix=[1 0 0; 0 1 0; 0 0 1]
  X2 : sm_lib/Body Elements/Solid  InertiaType=Custom  Mass=X2.m  MassUnits=kg  CenterOfMass=X2.cm  CenterOfMassUnits=m  MomentsOfInertia=[1 1 1]  MomentsOfInertiaUnits=kg*m^2  ProductsOfInertia=[0 0 0]  ProductsOfInertiaUnits=kg*m^2  DensityBased=on  Density=1000  DensityUnits=kg/(m^3)  DoExposeReferenceFrame=on  SerializedFrames=<Frames/>  GraphicType=FromGeometry  MarkerShape=Sphere  MarkerSize=10  MarkerSizeUnits=m  GraphicVisPropType=SimpleVisualProperties  GraphicDiffuseColor=X2.rgb  GraphicSpecularColor=[0.5 0.5 0.5 1.0]  GraphicAmbientColor=[0.15 0.15 0.15 1.0]  GraphicEmissiveColor=[0.0 0.0 0.0 1.0]  GraphicShininess=75  GraphicOpacity=1.0  GeometryShape=GeneralExtrusion  RectangleSize=[1 1]  RectangleSizeUnits=m  BrickDimensions=[1 1 1]  BrickDimensionUnits=m  CylinderRadius=1  CylinderRadiusUnits=m  CylinderLength=1  CylinderLengthUnits=m  SphereRadius=1  SphereRadiusUnits=m  EllipsoidRadii=[1 1 1]  EllipsoidRadiiUnits=m  ExtrusionCrossSection=X2.c  ExtrusionCrossSectionUnits=m  ExtrusionLength=X1.l  ExtrusionLengthUnits=m  PolygonNumSides=3  PolygonOuterRadius=1  PolygonOuterRadiusUnits=m  ExtGeomFileType=STEP  ExtGeomFileUnits=m  RevolutionCrossSection=[1 1; 1 -1; 2 -1; 2 1]  RevolutionCrossSectionUnits=m  RevolutionExtent=Full  RevolutionAngle=180  RevolutionAngleUnits=deg
  to X2 - Primastic : sm_lib/Frames and Transforms/Rigid Transform  TranslationMethod=Cartesian  TranslationStandardOffset=0  TranslationLengthUnit=m  TranslationStandardAxis=+Z  TranslationCartesianOffset=X2.pos  TranslationROffset=0  TranslationROffsetUnits=m  TranslationZOffset=0  TranslationZOffsetUnits=m  TranslationThetaOffset=0  TranslationThetaOffsetUnits=deg  RotationMethod=StandardAxis  RotationAngleUnits=deg  RotationStandardAxis=+Y  RotationAngle=90  RotationArbitraryAxis=[0 0 1]  FollAlignAxisA=+X  BaseAlignAxisA=+Y  FollAlignAxisB=+Y  BaseAlignAxisB=+Z  RotationSequenceAxes=FollowerAxes  RotationSequence=XYX  RotationSequenceAngles=[0 0 0]  RotationSequenceAnglesUnits=deg  RotationMatrix=[1 0 0; 0 1 0; 0 0 1]
  to X2v1 : PMIOPort  Port=1  Side=Right
  from X1 : PMIOPort  Port=2  Side=Left
  X2v : Outport
  wires:
  PS-Simulink Converter1/1 -> X2v/1
  connections:
  from X1/RConn1 -- to X2 - Primastic/LConn1
  to X2v1/RConn1 -- Cylinder Joint2/LConn2
  to X2 - Primastic/RConn1 -- Cylinder Joint2/LConn1
  PS-Simulink Converter1/LConn1 -- Cylinder Joint2/RConn2
  Rigid Transform1/RConn1 -- X2/RConn1
  Rigid Transform1/LConn1 -- Cylinder Joint2/RConn1

== system Final_IHA_2706_2015a/hydraulics/Cylinder1/Cylinder1/Chamber A ==
  Q_in : Inport
  " V" : Inport  Port=2
  " dV/dt" : Inport  Port=3
  " B" : Inport  Port=4
  Integrator : Integrator  InitialCondition=pinitial  AbsoluteTolerance=10
  Product : Product  Inputs=*/*  SaturateOnIntegerOverflow=on  InputSameDT=on  OutDataTypeStr=Inherit: Same as first input
  Saturation : Saturate  UpperLimit=inf  LowerLimit=0
  Sum : Sum  Inputs=+-  SaturateOnIntegerOverflow=on  InputSameDT=on  OutDataTypeStr=Inherit: Same as first input
  p : Outport
  wires:
  Sum/1 -> Product/1
  " dV/dt"/1 -> Sum/2
  Q_in/1 -> Sum/1
  " B"/1 -> Product/3
  " V"/1 -> Product/2
  Saturation/1 -> p/1
  Integrator/1 -> Saturation/1
  Product/1 -> Integrator/1

== system Final_IHA_2706_2015a/hydraulics/Cylinder1/Cylinder1/Chamber B ==
  Q_in : Inport
  " V" : Inport  Port=2
  " dV/dt" : Inport  Port=3
  " B" : Inport  Port=4
  Integrator : Integrator  InitialCondition=pinitial  AbsoluteTolerance=10
  Product : Product  Inputs=*/*  SaturateOnIntegerOverflow=on  InputSameDT=on  OutDataTypeStr=Inherit: Same as first input
  Saturation : Saturate  UpperLimit=inf  LowerLimit=0
  Sum : Sum  Inputs=+-  SaturateOnIntegerOverflow=on  InputSameDT=on  OutDataTypeStr=Inherit: Same as first input
  p : Outport
  wires:
  Sum/1 -> Product/1
  " dV/dt"/1 -> Sum/2
  Q_in/1 -> Sum/1
  " B"/1 -> Product/3
  " V"/1 -> Product/2
  Saturation/1 -> p/1
  Integrator/1 -> Saturation/1
  Product/1 -> Integrator/1

== system Final_IHA_2706_2015a/hydraulics/Cylinder1/Valve System1/Flow paths ==
  av_PA : Inport
  av_BT : Inport  Port=2
  av_PB : Inport  Port=3
  av_AT : Inport  Port=4
  p_A : Inport  Port=5
  p_B : Inport  Port=6
  p_S : Inport  Port=7
  "p_T " : Inport  Port=8
  Add{,1..3} (4 alike) : Sum
  Orifice AT : Subsystem  mask(Hydraulic){QN=Valve.AT.QN, dpN=Valve.PA.dpN, ptr=Valve.ptr}
      mask prompts: QN "Nominal Flow [m^3/s] :"; dpN "Nominal Pressure Difference [Pa] :"; ptr "Transition Pressure [Pa] :"
      mask help:
      | Implements numerically robust turbulent flow
      | equation. Polynomial flow equation is used
      | when abs(dp) < Transition Pressure.
      mask init:
      | K = QN/(sqrt(dpN));
      mask Help: eval('hydlibdoc(''orificedoc'')')
  Orifice BT : Subsystem  mask(Hydraulic){QN=Valve.BT.QN, dpN=Valve.PA.dpN, ptr=Valve.ptr}
      mask prompts: QN "Nominal Flow [m^3/s] :"; dpN "Nominal Pressure Difference [Pa] :"; ptr "Transition Pressure [Pa] :"
      mask help:
      | Implements numerically robust turbulent flow
      | equation. Polynomial flow equation is used
      | when abs(dp) < Transition Pressure.
      mask init:
      | K = QN/(sqrt(dpN));
      mask Help: eval('hydlibdoc(''orificedoc'')')
  Orifice PA : Subsystem  mask(Hydraulic){QN=Valve.PA.QN, dpN=Valve.PA.dpN, ptr=Valve.ptr}
      mask prompts: QN "Nominal Flow [m^3/s] :"; dpN "Nominal Pressure Difference [Pa] :"; ptr "Transition Pressure [Pa] :"
      mask help:
      | Implements numerically robust turbulent flow
      | equation. Polynomial flow equation is used
      | when abs(dp) < Transition Pressure.
      mask init:
      | K = QN/(sqrt(dpN));
      mask Help: eval('hydlibdoc(''orificedoc'')')
  Orifice PB : Subsystem  mask(Hydraulic){QN=Valve.PB.QN, dpN=Valve.PA.dpN, ptr=Valve.ptr}
      mask prompts: QN "Nominal Flow [m^3/s] :"; dpN "Nominal Pressure Difference [Pa] :"; ptr "Transition Pressure [Pa] :"
      mask help:
      | Implements numerically robust turbulent flow
      | equation. Polynomial flow equation is used
      | when abs(dp) < Transition Pressure.
      mask init:
      | K = QN/(sqrt(dpN));
      mask Help: eval('hydlibdoc(''orificedoc'')')
  Q_A : Outport
  Q_B : Outport  Port=2
  Q_P : Outport  Port=3
  Q_T : Outport  Port=4
  wires:
  p_A/1 -> Orifice AT/1(p_A), Orifice PA/2(p_A)
  p_S/1 -> Orifice PB/2(p_P), Orifice PA/1(p_P)
  "p_T "/1 -> Orifice BT/1(p_T), Orifice AT/2(p_T)
  p_B/1 -> Orifice PB/1(p_B), Orifice BT/2(p_B)
  av_PA/1 -> Orifice PA/3(u)
  av_BT/1 -> Orifice BT/3(u)
  av_AT/1 -> Orifice AT/3(u)
  av_PB/1 -> Orifice PB/3(u)
  Orifice PA/2(Q_A) -> Add/1
  Orifice AT/1(Q_A) -> Add/2
  Add/1 -> Q_A/1
  Orifice AT/2(Q_T) -> Add1/1
  Orifice BT/1(Q_T) -> Add1/2
  Add1/1 -> Q_T/1
  Orifice BT/2(Q_B) -> Add2/1
  Orifice PB/1(Q_B) -> Add2/2
  Add2/1 -> Q_B/1
  Add3/1 -> Q_P/1
  Orifice PA/1(Q_P) -> Add3/1
  Orifice PB/2(Q_P) -> Add3/2

== system Final_IHA_2706_2015a/hydraulics/Cylinder1/Valve System1/Relative openings ==
  Spool_position : Inport
  1-D Lookup Table : Lookup_n-D  NumberOfTableDimensions=1  BreakpointsForDimension1=Q_PA_break  Table=Q_PA_look  InternalRulePriority=Speed  RndMeth=Simplest  InputSameDT=on
  1-D Lookup Table1 : Lookup_n-D  NumberOfTableDimensions=1  BreakpointsForDimension1=Q_PB_break  Table=Q_PB_look  InternalRulePriority=Speed  RndMeth=Simplest  InputSameDT=on
  1-D Lookup Table2 : Lookup_n-D  NumberOfTableDimensions=1  BreakpointsForDimension1=Q_BT_break  Table=Q_BT_look  InternalRulePriority=Speed  RndMeth=Simplest  InputSameDT=on
  1-D Lookup Table3 : Lookup_n-D  NumberOfTableDimensions=1  BreakpointsForDimension1=Q_AT_break  Table=Q_AT_look  InternalRulePriority=Speed  RndMeth=Simplest  InputSameDT=on
  av_PA : Outport
  av_PB : Outport  Port=2
  av_BT : Outport  Port=3
  av_AT : Outport  Port=4
  wires:
  1-D Lookup Table3/1 -> av_AT/1
  1-D Lookup Table/1 -> av_PA/1
  1-D Lookup Table2/1 -> av_BT/1
  1-D Lookup Table1/1 -> av_PB/1
  Spool_position/1 -> 1-D Lookup Table3/1, 1-D Lookup Table1/1, 1-D Lookup Table2/1, 1-D Lookup Table/1

== system Final_IHA_2706_2015a/hydraulics/Cylinder1/Valve System1/Valve Dynamics ==
  Control [-1....1] : Inport
  Saturation1 : Saturate  UpperLimit=1  LowerLimit=-1
  Transfer Fcn1 : TransferFcn  Numerator=[q^2]  Denominator=[1 2*t*q q^2]
  Transport Delay1 : TransportDelay  DelayTime=Valve.delay
  Spool Position [-1....1] : Outport
  wires:
  Transport Delay1/1 -> Transfer Fcn1/1
  Transfer Fcn1/1 -> Saturation1/1
  Control [-1....1]/1 -> Transport Delay1/1
  Saturation1/1 -> Spool Position [-1....1]/1

== system Final_IHA_2706_2015a/hydraulics/Cylinder2/Cylinder2/Chamber A ==
  Q_in : Inport
  " V" : Inport  Port=2
  " dV/dt" : Inport  Port=3
  " B" : Inport  Port=4
  Integrator : Integrator  InitialCondition=pinitial  AbsoluteTolerance=10
  Product : Product  Inputs=*/*  SaturateOnIntegerOverflow=on  InputSameDT=on  OutDataTypeStr=Inherit: Same as first input
  Saturation : Saturate  UpperLimit=inf  LowerLimit=0
  Sum : Sum  Inputs=+-  SaturateOnIntegerOverflow=on  InputSameDT=on  OutDataTypeStr=Inherit: Same as first input
  p : Outport
  wires:
  Product/1 -> Integrator/1
  Integrator/1 -> Saturation/1
  Saturation/1 -> p/1
  " V"/1 -> Product/2
  " B"/1 -> Product/3
  Q_in/1 -> Sum/1
  " dV/dt"/1 -> Sum/2
  Sum/1 -> Product/1

== system Final_IHA_2706_2015a/hydraulics/Cylinder2/Cylinder2/Chamber B ==
  Q_in : Inport
  " V" : Inport  Port=2
  " dV/dt" : Inport  Port=3
  " B" : Inport  Port=4
  Integrator : Integrator  InitialCondition=pinitial  AbsoluteTolerance=10
  Product : Product  Inputs=*/*  SaturateOnIntegerOverflow=on  InputSameDT=on  OutDataTypeStr=Inherit: Same as first input
  Saturation : Saturate  UpperLimit=inf  LowerLimit=0
  Sum : Sum  Inputs=+-  SaturateOnIntegerOverflow=on  InputSameDT=on  OutDataTypeStr=Inherit: Same as first input
  p : Outport
  wires:
  Product/1 -> Integrator/1
  Integrator/1 -> Saturation/1
  Saturation/1 -> p/1
  " V"/1 -> Product/2
  " B"/1 -> Product/3
  Q_in/1 -> Sum/1
  " dV/dt"/1 -> Sum/2
  Sum/1 -> Product/1

== system Final_IHA_2706_2015a/hydraulics/Cylinder2/Valve System2/Flow paths ==
  av_PA : Inport
  av_BT : Inport  Port=2
  av_PB : Inport  Port=3
  av_AT : Inport  Port=4
  p_A : Inport  Port=5
  p_B : Inport  Port=6
  p_S : Inport  Port=7
  "p_T " : Inport  Port=8
  Add{,1..3} (4 alike) : Sum
  Orifice AT : Subsystem  mask(Hydraulic){QN=Valve2.AT.QN, dpN=Valve2.PA.dpN, ptr=Valve.ptr}
      mask prompts: QN "Nominal Flow [m^3/s] :"; dpN "Nominal Pressure Difference [Pa] :"; ptr "Transition Pressure [Pa] :"
      mask help:
      | Implements numerically robust turbulent flow
      | equation. Polynomial flow equation is used
      | when abs(dp) < Transition Pressure.
      mask init:
      | K = QN/(sqrt(dpN));
      mask Help: eval('hydlibdoc(''orificedoc'')')
  Orifice BT : Subsystem  mask(Hydraulic){QN=Valve2.BT.QN, dpN=Valve2.PA.dpN, ptr=Valve.ptr}
      mask prompts: QN "Nominal Flow [m^3/s] :"; dpN "Nominal Pressure Difference [Pa] :"; ptr "Transition Pressure [Pa] :"
      mask help:
      | Implements numerically robust turbulent flow
      | equation. Polynomial flow equation is used
      | when abs(dp) < Transition Pressure.
      mask init:
      | K = QN/(sqrt(dpN));
      mask Help: eval('hydlibdoc(''orificedoc'')')
  Orifice PA : Subsystem  mask(Hydraulic){QN=Valve2.PA.QN, dpN=Valve2.PA.dpN, ptr=Valve.ptr}
      mask prompts: QN "Nominal Flow [m^3/s] :"; dpN "Nominal Pressure Difference [Pa] :"; ptr "Transition Pressure [Pa] :"
      mask help:
      | Implements numerically robust turbulent flow
      | equation. Polynomial flow equation is used
      | when abs(dp) < Transition Pressure.
      mask init:
      | K = QN/(sqrt(dpN));
      mask Help: eval('hydlibdoc(''orificedoc'')')
  Orifice PB : Subsystem  mask(Hydraulic){QN=Valve2.PB.QN, dpN=Valve2.PA.dpN, ptr=Valve.ptr}
      mask prompts: QN "Nominal Flow [m^3/s] :"; dpN "Nominal Pressure Difference [Pa] :"; ptr "Transition Pressure [Pa] :"
      mask help:
      | Implements numerically robust turbulent flow
      | equation. Polynomial flow equation is used
      | when abs(dp) < Transition Pressure.
      mask init:
      | K = QN/(sqrt(dpN));
      mask Help: eval('hydlibdoc(''orificedoc'')')
  Q_A : Outport
  Q_B : Outport  Port=2
  Q_P : Outport  Port=3
  Q_T : Outport  Port=4
  wires:
  Orifice PB/2(Q_P) -> Add3/2
  Orifice PA/1(Q_P) -> Add3/1
  Add3/1 -> Q_P/1
  Add2/1 -> Q_B/1
  Orifice PB/1(Q_B) -> Add2/2
  Orifice BT/2(Q_B) -> Add2/1
  Add1/1 -> Q_T/1
  Orifice BT/1(Q_T) -> Add1/2
  Orifice AT/2(Q_T) -> Add1/1
  Add/1 -> Q_A/1
  Orifice AT/1(Q_A) -> Add/2
  Orifice PA/2(Q_A) -> Add/1
  av_PB/1 -> Orifice PB/3(u)
  av_AT/1 -> Orifice AT/3(u)
  av_BT/1 -> Orifice BT/3(u)
  av_PA/1 -> Orifice PA/3(u)
  p_B/1 -> Orifice BT/2(p_B), Orifice PB/1(p_B)
  "p_T "/1 -> Orifice AT/2(p_T), Orifice BT/1(p_T)
  p_S/1 -> Orifice PA/1(p_P), Orifice PB/2(p_P)
  p_A/1 -> Orifice PA/2(p_A), Orifice AT/1(p_A)

== system Final_IHA_2706_2015a/hydraulics/Cylinder2/Valve System2/Relative openings ==
  Spool_position : Inport
  1-D Lookup Table : Lookup_n-D  NumberOfTableDimensions=1  BreakpointsForDimension1=Q_PA_break  Table=Q_PA_look  InternalRulePriority=Speed  RndMeth=Simplest  InputSameDT=on
  1-D Lookup Table1 : Lookup_n-D  NumberOfTableDimensions=1  BreakpointsForDimension1=Q_PB_break  Table=Q_PB_look  InternalRulePriority=Speed  RndMeth=Simplest  InputSameDT=on
  1-D Lookup Table2 : Lookup_n-D  NumberOfTableDimensions=1  BreakpointsForDimension1=Q_BT_break  Table=Q_BT_look  InternalRulePriority=Speed  RndMeth=Simplest  InputSameDT=on
  1-D Lookup Table3 : Lookup_n-D  NumberOfTableDimensions=1  BreakpointsForDimension1=Q_AT_break  Table=Q_AT_look  InternalRulePriority=Speed  RndMeth=Simplest  InputSameDT=on
  av_PA : Outport
  av_PB : Outport  Port=2
  av_BT : Outport  Port=3
  av_AT : Outport  Port=4
  wires:
  Spool_position/1 -> 1-D Lookup Table/1, 1-D Lookup Table2/1, 1-D Lookup Table1/1, 1-D Lookup Table3/1
  1-D Lookup Table1/1 -> av_PB/1
  1-D Lookup Table2/1 -> av_BT/1
  1-D Lookup Table/1 -> av_PA/1
  1-D Lookup Table3/1 -> av_AT/1

== system Final_IHA_2706_2015a/hydraulics/Cylinder2/Valve System2/Valve Dynamics ==
  Control [-1....1] : Inport
  Saturation1 : Saturate  UpperLimit=1  LowerLimit=-1
  Transfer Fcn1 : TransferFcn  Numerator=[q^2]  Denominator=[1 2*t*q q^2]
  Transport Delay1 : TransportDelay  DelayTime=Valve.delay
  Spool Position [-1....1] : Outport
  wires:
  Saturation1/1 -> Spool Position [-1....1]/1
  Control [-1....1]/1 -> Transport Delay1/1
  Transfer Fcn1/1 -> Saturation1/1
  Transport Delay1/1 -> Transfer Fcn1/1

== system Final_IHA_2706_2015a/hydraulics/Cylinder3/Cylinder3/Chamber A ==
  Q_in : Inport
  " V" : Inport  Port=2
  " dV/dt" : Inport  Port=3
  " B" : Inport  Port=4
  Integrator : Integrator  InitialCondition=pinitial  AbsoluteTolerance=10
  Product : Product  Inputs=*/*  SaturateOnIntegerOverflow=on  InputSameDT=on  OutDataTypeStr=Inherit: Same as first input
  Saturation : Saturate  UpperLimit=inf  LowerLimit=0
  Sum : Sum  Inputs=+-  SaturateOnIntegerOverflow=on  InputSameDT=on  OutDataTypeStr=Inherit: Same as first input
  p : Outport
  wires:
  Sum/1 -> Product/1
  " dV/dt"/1 -> Sum/2
  Q_in/1 -> Sum/1
  " B"/1 -> Product/3
  " V"/1 -> Product/2
  Saturation/1 -> p/1
  Integrator/1 -> Saturation/1
  Product/1 -> Integrator/1

== system Final_IHA_2706_2015a/hydraulics/Cylinder3/Cylinder3/Chamber B ==
  Q_in : Inport
  " V" : Inport  Port=2
  " dV/dt" : Inport  Port=3
  " B" : Inport  Port=4
  Integrator : Integrator  InitialCondition=pinitial  AbsoluteTolerance=10
  Product : Product  Inputs=*/*  SaturateOnIntegerOverflow=on  InputSameDT=on  OutDataTypeStr=Inherit: Same as first input
  Saturation : Saturate  UpperLimit=inf  LowerLimit=0
  Sum : Sum  Inputs=+-  SaturateOnIntegerOverflow=on  InputSameDT=on  OutDataTypeStr=Inherit: Same as first input
  p : Outport
  wires:
  Sum/1 -> Product/1
  " dV/dt"/1 -> Sum/2
  Q_in/1 -> Sum/1
  " B"/1 -> Product/3
  " V"/1 -> Product/2
  Saturation/1 -> p/1
  Integrator/1 -> Saturation/1
  Product/1 -> Integrator/1

== system Final_IHA_2706_2015a/hydraulics/Cylinder3/Valve System3/Flow paths ==
  av_PA : Inport
  av_BT : Inport  Port=2
  av_PB : Inport  Port=3
  av_AT : Inport  Port=4
  p_A : Inport  Port=5
  p_B : Inport  Port=6
  p_S : Inport  Port=7
  "p_T " : Inport  Port=8
  Add{,1..3} (4 alike) : Sum
  Orifice AT : Subsystem  mask(Hydraulic){QN=Valve3.AT.QN, dpN=Valve3.PA.dpN, ptr=Valve.ptr}
      mask prompts: QN "Nominal Flow [m^3/s] :"; dpN "Nominal Pressure Difference [Pa] :"; ptr "Transition Pressure [Pa] :"
      mask help:
      | Implements numerically robust turbulent flow
      | equation. Polynomial flow equation is used
      | when abs(dp) < Transition Pressure.
      mask init:
      | K = QN/(sqrt(dpN));
      mask Help: eval('hydlibdoc(''orificedoc'')')
  Orifice BT : Subsystem  mask(Hydraulic){QN=Valve3.BT.QN, dpN=Valve3.PA.dpN, ptr=Valve.ptr}
      mask prompts: QN "Nominal Flow [m^3/s] :"; dpN "Nominal Pressure Difference [Pa] :"; ptr "Transition Pressure [Pa] :"
      mask help:
      | Implements numerically robust turbulent flow
      | equation. Polynomial flow equation is used
      | when abs(dp) < Transition Pressure.
      mask init:
      | K = QN/(sqrt(dpN));
      mask Help: eval('hydlibdoc(''orificedoc'')')
  Orifice PA : Subsystem  mask(Hydraulic){QN=Valve3.PA.QN, dpN=Valve3.PA.dpN, ptr=Valve.ptr}
      mask prompts: QN "Nominal Flow [m^3/s] :"; dpN "Nominal Pressure Difference [Pa] :"; ptr "Transition Pressure [Pa] :"
      mask help:
      | Implements numerically robust turbulent flow
      | equation. Polynomial flow equation is used
      | when abs(dp) < Transition Pressure.
      mask init:
      | K = QN/(sqrt(dpN));
      mask Help: eval('hydlibdoc(''orificedoc'')')
  Orifice PB : Subsystem  mask(Hydraulic){QN=Valve3.PB.QN, dpN=Valve3.PA.dpN, ptr=Valve.ptr}
      mask prompts: QN "Nominal Flow [m^3/s] :"; dpN "Nominal Pressure Difference [Pa] :"; ptr "Transition Pressure [Pa] :"
      mask help:
      | Implements numerically robust turbulent flow
      | equation. Polynomial flow equation is used
      | when abs(dp) < Transition Pressure.
      mask init:
      | K = QN/(sqrt(dpN));
      mask Help: eval('hydlibdoc(''orificedoc'')')
  Q_A : Outport
  Q_B : Outport  Port=2
  Q_P : Outport  Port=3
  Q_T : Outport  Port=4
  wires:
  p_A/1 -> Orifice AT/1(p_A), Orifice PA/2(p_A)
  p_S/1 -> Orifice PB/2(p_P), Orifice PA/1(p_P)
  "p_T "/1 -> Orifice BT/1(p_T), Orifice AT/2(p_T)
  p_B/1 -> Orifice PB/1(p_B), Orifice BT/2(p_B)
  av_PA/1 -> Orifice PA/3(u)
  av_BT/1 -> Orifice BT/3(u)
  av_AT/1 -> Orifice AT/3(u)
  av_PB/1 -> Orifice PB/3(u)
  Orifice PA/2(Q_A) -> Add/1
  Orifice AT/1(Q_A) -> Add/2
  Add/1 -> Q_A/1
  Orifice AT/2(Q_T) -> Add1/1
  Orifice BT/1(Q_T) -> Add1/2
  Add1/1 -> Q_T/1
  Orifice BT/2(Q_B) -> Add2/1
  Orifice PB/1(Q_B) -> Add2/2
  Add2/1 -> Q_B/1
  Add3/1 -> Q_P/1
  Orifice PA/1(Q_P) -> Add3/1
  Orifice PB/2(Q_P) -> Add3/2
